simulink model "infant_respiratory_model"  (R2024a)
settings: Solver=ode15s  StartTime=0.0  StopTime=1000  MaxStep=0.05  RelTol=1e-3
settings Model: Creator=ASUS  LastModifiedBy=ASUS

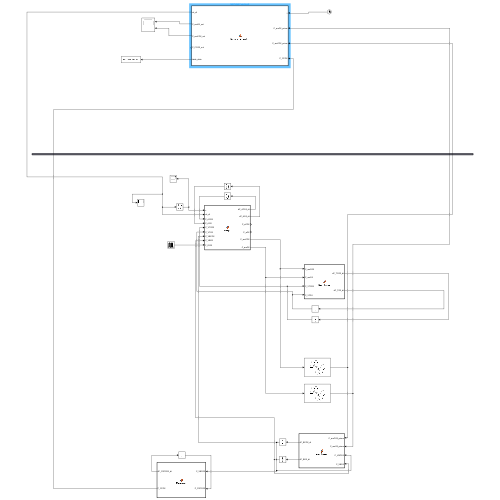
[thumbnail: Simulink's stored preview of the top-level diagram]
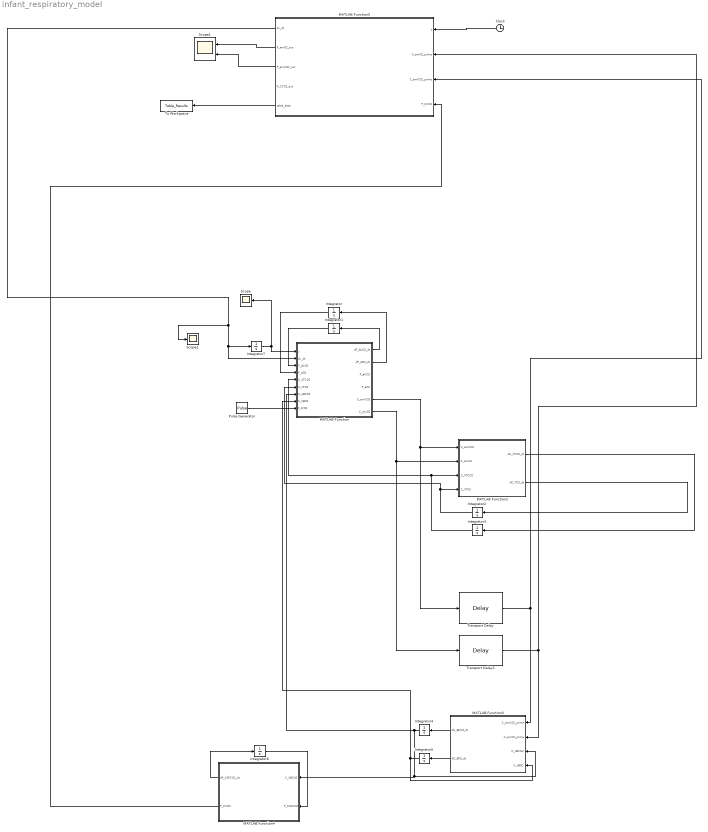
== system infant_respiratory_model ==
  Clock : Clock
  Integrator : Integrator  InitialCondition=100  LimitOutput=on  LowerSaturationLimit=0
  Integrator1 : Integrator  InitialCondition=40  LimitOutput=on  LowerSaturationLimit=0
  Integrator2 : Integrator  InitialCondition=0.19
  Integrator3 : Integrator  InitialCondition=0.64
  Integrator4 : Integrator  InitialCondition=0.64
  Integrator5 : Integrator  InitialCondition=0.19
  Integrator6 : Integrator  InitialCondition=45
  Integrator7 : Integrator  InitialCondition=0.08  LimitOutput=on  LowerSaturationLimit=0.08
  MATLAB Function : MATLAB Function  TreatAsAtomicUnit=on
  MATLAB Function2 : MATLAB Function  TreatAsAtomicUnit=on
  MATLAB Function3 : MATLAB Function  TreatAsAtomicUnit=on
  MATLAB Function4 : MATLAB Function  TreatAsAtomicUnit=on
  MATLAB Function5 : MATLAB Function  TreatAsAtomicUnit=on
  Pulse Generator : DiscretePulseGenerator  PulseType=Time based  Amplitude=0.05  Period=1000  PulseWidth=50  PhaseDelay=500
  Scope : Scope
  Scope1 : Scope  NumInputPorts=2
  Scope2 : Scope
  To Workspace : ToWorkspace  VariableName=Table_Results  SampleTime=-1
  Transport Delay : TransportDelay  DelayTime=4  InitialOutput=0.64  BufferSize=10240
  Transport Delay1 : TransportDelay  DelayTime=4  InitialOutput=0.19  BufferSize=10240
  wires:
  MATLAB Function/1(dP_ACO2_dt) -> Integrator1/1
  MATLAB Function/2(dP_AO2_dt) -> Integrator/1
  Integrator1/1 -> MATLAB Function/3(P_ACO2)
  Integrator/1 -> MATLAB Function/4(P_AO2)
  MATLAB Function/5(C_amCO2) -> Transport Delay/1, MATLAB Function2/1(C_amCO2)
  MATLAB Function/6(C_amO2) -> Transport Delay1/1, MATLAB Function2/2(C_amO2)
  MATLAB Function2/2(dC_TO2_dt) -> Integrator2/1
  MATLAB Function2/1(dC_TCO2_dt) -> Integrator3/1
  Integrator2/1 -> MATLAB Function/6(C_VTO2), MATLAB Function2/4(C_VTO2)
  Integrator3/1 -> MATLAB Function/5(C_VTCO2), MATLAB Function2/3(C_VTCO2)
  Transport Delay/1 -> MATLAB Function5/3(C_amCO2_prime), MATLAB Function3/1(C_amCO2_prime)
  Transport Delay1/1 -> MATLAB Function5/2(C_amO2_prime), MATLAB Function3/2(C_amO2_prime)
  MATLAB Function3/2(dC_BO2_dt) -> Integrator5/1
  MATLAB Function3/1(dC_BCO2_dt) -> Integrator4/1
  Integrator5/1 -> MATLAB Function/8(C_VBO2), MATLAB Function3/4(C_VBO2)
  Integrator4/1 -> MATLAB Function4/1(C_VBCO2), MATLAB Function3/3(C_VBCO2), MATLAB Function/7(C_VBCO2)
  MATLAB Function4/1(dP_CSFCO2_dt) -> Integrator6/1
  Integrator6/1 -> MATLAB Function4/2(P_CSFCO2)
  Clock/1 -> MATLAB Function5/1(t)
  MATLAB Function4/2(P_CCO2) -> MATLAB Function5/4(P_CCO2)
  MATLAB Function5/1(dv_dt) -> Scope2/1, MATLAB Function/2(dv_dt), Integrator7/1
  Integrator7/1 -> Scope/1, MATLAB Function/1(v)
  MATLAB Function5/2(P_amO2_out) -> Scope1/1
  MATLAB Function5/3(P_amCO2_out) -> Scope1/2
  Pulse Generator/1 -> MATLAB Function/9(F_ICO2)
  MATLAB Function5/5(table_data) -> To Workspace/1

== matlab function infant_respiratory_model/MATLAB Function ==
  data: v input; dP_ACO2_dt output; dv_dt input; P_ACO2 input; P_AO2 input; C_VTCO2 input; C_VTO2 input; C_VBCO2 input; C_VBO2 input; dP_AO2_dt output; P_aCO2 output; P_aO2 output; C_amCO2 output; C_amO2 output; F_ICO2 input
function [dP_ACO2_dt, dP_AO2_dt, P_aCO2, P_aO2, C_amCO2, C_amO2] = Lungs(v, dv_dt, P_ACO2, P_AO2, C_VTCO2, C_VTO2, C_VBCO2, C_VBO2,F_ICO2)
    
    % --- Constants ---
    P_b = 760;          
    alpha = 0.1;        
    K = 20;             
    Q = 13.13e-3;       
    Q_T = 9.8e-3;       
    Q_B = 3.33e-3;      
    K3 = 0.016;  
    K4 = 0.2;    
    K5 = 0.046;  
    
    F_IO2 = 0.21;       
            
    
    P_IO2 = F_IO2 * (P_b - 47);
    P_ICO2 = F_ICO2 * (P_b - 47);

    % --- 1. Ventilation (Eqs 1 & 2 part 1) ---
    if dv_dt >= 0
        G1 = ((P_ACO2 - P_ICO2) * dv_dt) / (P_b - 47);
        G2 = ((P_AO2 - P_IO2) * dv_dt) / (P_b - 47);
    else
        G1 = 0;
        G2 = 0;
    end

    % --- 2. Arterial Pressures (Eqs 3 & 4) ---
    P_aCO2 = P_ACO2;
    P_aO2  = P_AO2 - K;

    % --- 3. Blood Gas Conversions (Eqs 15 & 16) --- 
    C_aCO2 = K3 * P_aCO2;
    C_aO2 = K4 * (1 - exp(-K5 * P_aO2))^2;

    % --- 4. Alveolar Pressure Derivatives (Eqs 1 & 2 part 2) ---
    term_CO2 = (C_VTCO2 - C_aCO2)*(1 - alpha)*Q_T + (C_VBCO2 - C_aCO2)*(1 - alpha)*Q_B;
    term_O2  = (C_VTO2 - C_aO2)*(1 - alpha)*Q_T  + (C_VBO2 - C_aO2)*(1 - alpha)*Q_B;

    dP_ACO2_dt = ((P_b - 47) / v) * (term_CO2 - G1);
    dP_AO2_dt  = ((P_b - 47) / v) * (term_O2 - G2);

    % --- 5. Mixed Arterial Concentrations (Eqs 5 & 6) ---
    C_amCO2 = (1 - alpha)*C_aCO2 + (alpha*Q_T/Q)*C_VTCO2 + (alpha*Q_B/Q)*C_VBCO2;
    C_amO2  = (1 - alpha)*C_aO2  + (alpha*Q_T/Q)*C_VTO2  + (alpha*Q_B/Q)*C_VBO2;
end

== matlab function infant_respiratory_model/MATLAB Function2 ==
  data: C_amCO2 input; dC_TCO2_dt output; C_amO2 input; C_VTCO2 input; C_VTO2 input; dC_TO2_dt output
function [dC_TCO2_dt, dC_TO2_dt] = BodyTissue(C_amCO2, C_amO2, C_VTCO2, C_VTO2)
    
    % --- Constants from Appendix ---
    Q_T = 9.8e-3;           % (l/s)
    MR_TCO2 = 1.625e-4;     % (l/s)
    MR_TO2 = 1.902e-4;      % (l/s)
    S_T = 0.9;              % (l)

    % --- Equations ---
    dC_TCO2_dt = (C_amCO2 * Q_T + MR_TCO2 - C_VTCO2 * Q_T) / S_T;
    dC_TO2_dt  = (C_amO2 * Q_T - MR_TO2 - C_VTO2 * Q_T) / S_T;
end

== matlab function infant_respiratory_model/MATLAB Function3 ==
  data: C_amCO2_prime input; dC_BCO2_dt output; C_amO2_prime input; C_VBCO2 input; C_VBO2 input; dC_BO2_dt output
function [dC_BCO2_dt, dC_BO2_dt] = BrainTissue(C_amCO2_prime, C_amO2_prime, C_VBCO2, C_VBO2)
    
    % --- Constants from Appendix ---
    Q_B = 3.33e-3;          % (l/s)
    MR_BCO2 = 2.6154e-4;    % (l/s)
    MR_BO2 = 2.78697e-4;    % (l/s)
    S_B = 0.067;            % (l)

    % --- Equations ---
    dC_BCO2_dt = (C_amCO2_prime * Q_B + MR_BCO2 - C_VBCO2 * Q_B) / S_B;
    dC_BO2_dt  = (C_amO2_prime * Q_B - MR_BO2 - C_VBO2 * Q_B) / S_B;
end

== matlab function infant_respiratory_model/MATLAB Function4 ==
  data: C_VBCO2 input; dP_CSFCO2_dt output; P_CSFCO2 input; P_CCO2 output
function [dP_CSFCO2_dt, P_CCO2] = Receptors(C_VBCO2, P_CSFCO2)
    
    % --- Constants from Appendix ---
    Q_B = 3.33e-3;
    K1 = 346e3;
    K2 = 320;
    K3 = 0.016;
    d = 15e-3;

    % --- Equations ---
    P_VBCO2 = C_VBCO2 / K3;
    dP_CSFCO2_dt = (1 / K2) * (P_VBCO2 - P_CSFCO2);
    P_CCO2 = P_VBCO2 + (P_CSFCO2 - P_VBCO2) * exp(-d * sqrt(Q_B * K1));
end

== matlab function infant_respiratory_model/MATLAB Function5 ==
  settings: updateMethod=DISCRETE  sampleTime=0.01
  data: t input; C_amO2_prime input; dv_dt output; C_amCO2_prime input; P_CCO2 input; P_amO2_out output; P_amCO2_out output; P_CCO2_out output; table_data output
function [dv_dt, P_amO2_out, P_amCO2_out, P_CCO2_out ,table_data] = Discrete_Controller(t, C_amO2_prime, C_amCO2_prime, P_CCO2)
    
    % --- Constants ---
    beta = 17.1756;
    V_A_rest = 0.491 / 60;   
    K3 = 0.016; 
    K4 = 0.2; 
    K5 = 0.046;
    mu = 1.0;           % Test Condition (1.0, 0.8, or 0.5)
    gamma = 91; 
    lambda = 60;

    % --- Persistent Variables ---
    persistent t_next t_prev
    persistent sum_PO2 sum_PCO2 sum_PCCO2
    persistent V_A_dot_hold f_hold ratio_hold t_start_breath 
    persistent mean_PO2_hold mean_PCO2_hold % <--- اضافه شدن حافظه برای میانگین گازها

    if isempty(t_next)
        f_hold = 0.5; 
        t_next = 1 / f_hold; 
        t_prev = 0;
        sum_PO2 = 0;
        sum_PCO2 = 0;
        sum_PCCO2 = 0;
        V_A_dot_hold = 0.0043; 
        ratio_hold = 1.0; 
        t_start_breath = 0; 
        mean_PO2_hold = 80; % مقدار اولیه میانگین اکسیژن
        mean_PCO2_hold = 40; % مقدار اولیه میانگین دی‌اکسید کربن
    end

    % ---------------------------------------------------------
    % 1. آشکارساز مقدار میانگین (Mean Value Detector)
    % ---------------------------------------------------------
    C_O2_safe = min(C_amO2_prime, 0.999 * K4); 
    C_O2_safe = max(C_O2_safe, 0);
    
    P_amO2_inst  = (-1/K5) * log(1 - sqrt(C_O2_safe / K4));
    P_amCO2_inst = max(C_amCO2_prime / K3, 0);

    dt = t - t_prev;
    if dt > 0
        sum_PO2   = sum_PO2 + (P_amO2_inst * dt);
        sum_PCO2  = sum_PCO2 + (P_amCO2_inst * dt);
        sum_PCCO2 = sum_PCCO2 + (P_CCO2 * dt);
    end
    t_prev = t;

    % ---------------------------------------------------------
    % 2. تولیدکننده پالس ساعت (Clock Pulse Generator)
    % ---------------------------------------------------------
    if t >= t_next 
        
        breath_duration = 1 / f_hold;
        mean_PO2  = sum_PO2 / breath_duration;
        mean_PCO2 = sum_PCO2 / breath_duration;
        mean_PCCO2 = sum_PCCO2 / breath_duration;

        mean_PO2_hold = mean_PO2;
        mean_PCO2_hold = mean_PCO2;

        sum_PO2 = 0;
        sum_PCO2 = 0;
        sum_PCCO2 = 0;

        % ---------------------------------------------------------
        % 3. کنترلر تهویه (Ventilation Controller)
        % ---------------------------------------------------------
        if mean_PO2 < 104
            F1 = 4.72e-9 * mu * (104 - mean_PO2)^4.9;
        else
            F1 = 0;
        end
        
        ratio = 0.2025 * mean_PCO2 + 0.2332 * mean_PCCO2 + F1 - beta;
        ratio_hold = ratio; 
        
        if ratio < 0
            V_A_dot_new = 0; 
        else
            V_A_dot_new = ratio * V_A_rest;
        end
        
        % ---------------------------------------------------------
        % 4. بهینه‌ساز فرکانس (Frequency Optimizer)
        % ---------------------------------------------------------
        V_D_new = 0.1698 * V_A_dot_new + 2.28e-3;
        num = -gamma * V_D_new + sqrt((gamma * V_D_new)^2 + 4 * gamma * lambda * pi^2 * V_D_new * V_A_dot_new);
        den = 2 * pi^2 * lambda * V_D_new;
        f_new = num / den;
        
        V_A_dot_hold = V_A_dot_new;
        if f_new > 0
            f_hold = f_new;
        else
            f_hold = 0.5; 
        end
        
        t_start_breath = t;
        t_next = t + (1 / f_hold);
    end

    % ---------------------------------------------------------
    % 5. تخصیص خروجی‌ها
    % ---------------------------------------------------------
    current_breath_time = t - t_start_breath; 
    
    dv_dt = pi * V_A_dot_hold * sin(2 * pi * f_hold * current_breath_time);
    
    P_amO2_out  = mean_PO2_hold;
    P_amCO2_out = mean_PCO2_hold;
    P_CCO2_out  = P_CCO2; 


    % ---------------------------------------------------------
    % 6. خروجی مخصوص استخراج جدول مقاله (Table I)
    % ---------------------------------------------------------
    % تبدیل واحدها به دقیقه (ضرب در 60)
    % 1. محاسبه حجم فضای مرده در این نفس
    V_D_hold = 0.1698 * V_A_dot_hold + 2.28e-3; 
    
    % 2. محاسبه تهویه کل (دهانی)
    V_E_dot_hold = V_A_dot_hold + (f_hold * V_D_hold);
    V_A_min = V_A_dot_hold * 60;
    V_E_min = V_E_dot_hold * 60;
    f_min   = f_hold * 60;
    
    % بسته‌بندی 7 متغیر جدول در یک آرایه
    % ترتیب: [PO2, PCO2, P_CCO2, V_A, V_D, V_E, f]
    table_data = [mean_PO2_hold, mean_PCO2_hold, P_CCO2, V_A_min, V_D_hold, V_E_min, f_min];

end
